simulink model "MOSSE_HDL_code_gen_final"  (Simulink 8.2)
settings: Solver=FixedStepDiscrete  SolverMode=SingleTasking  StartTime=0.0  StopTime=20*640*360  RelTol=1e-3
InitFcn:
  | %% DSPBuilder Start
  | alt_dspbuilder_update_model(bdroot)
  | %% DSPBuilder End
  | param
StopFcn:
  | % r = rcount.Data(:,:);
  | % w = wcount.Data(:,:);
  | % d = dout.Data(:,:);
  | % ir = read.Data(:,:);
  | % iw = write.Data(:,:);
  | % z = double([ir iw d r w]');
  | %logic_analyzer
values from neighbouring files (symbols this model uses):
  Gau = [4035 -3983 3832 -3589 3269 -2890 2472 -2039 1612 -1211 854 -553 ... (4096 elements, 1x4096)]    [Gauss_coeff.mat]    (also in param.m = reshape(conj(Gau'), 1, 4096))
undefined symbols (not defined in the file or in its folder): jet, psr, source_1, source_2, State_Machine, State_Transition_Table1, window_hann
libraries: allblocks_alteradspbuilder2 x182, hdldemolib x2, dspsigattribs x2, dspmtrx3 x2, visionsinks x1, visiontextngfix x1, dspvision x1
(part 1 of 3)
settings Model: FPTRunName=FPA_Reference  Creator=minimal  LastModifiedBy=Roma
settings DataIOCC: SignalLoggingSaveFormat=Dataset
settings OptimizationCC: ExpressionDepthLimit=128  OptimizeModelRefInitCode=on  LifeSpan=9
settings DebuggingCC: FcnCallInpInsideContextMsg=EnableAllAsError
settings HardwareCC: ProdHWDeviceType=ASIC/FPGA->ASIC/FPGA  TargetIntDivRoundTo=Zero  TargetEndianess=LittleEndian  TargetHWDeviceType=MATLAB Host  ProdEqTarget=off
settings RTWCC: SystemTargetFile=ert.tlc  TemplateMakefile=ert_default_tmf  Description=Embedded Coder  ProcessScript=ert_make_rtw_hook
settings CodeAppCC: IgnoreCustomStorageClasses=off
settings ERTTargetCC: CodeReplacementLibrary=ANSI_C  MultiwordLength=2048  GenerateSampleERTMain=on  ERTCustomFileTemplate=example_file_process.tlc  ConvertIfToSwitch=off  SuppressUnreachableDefaultCases=off

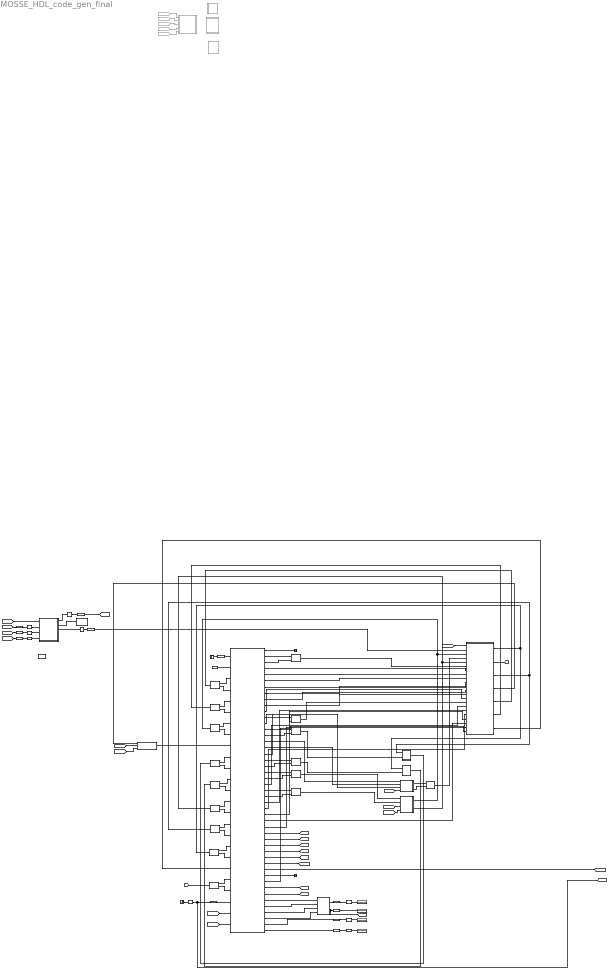
== system MOSSE_HDL_code_gen_final ==
  Complex to Real-Imag1 : allblocks_alteradspbuilder2/Complex to Real-Imag  BusType=Signed Integer  bwl=32  bwr=0  pipeline_display=0  allowFloatingPointOverride=on  logOutputs=off  logFile=E:\Project\AutoTracking\AutoTrack\Model\MOSSE_algorithm\MOSSE_simulink\tb_MOSSE_HDL_code_gen_final\MOSSE%5FHDL%5Fcode%5Fgen%5Ffinal_Complex+to+Real-Imag1%3A%3Aoutput%5Freal.fixedpointlog,E:\Project\AutoTracking\AutoTrack\Model\MOSSE_algorithm\MOSSE_simulink\tb_MOSSE_HDL_code_gen_final\MOSSE%5FHDL%5Fcode%5Fgen%5Ffinal_Complex+to+Real-Imag1%3A%3Aoutput%5Fimag.fixedpointlog,
  Complex to Real-Imag2 : allblocks_alteradspbuilder2/Complex to Real-Imag  BusType=Signed Integer  bwl=32  bwr=0  pipeline_display=0  allowFloatingPointOverride=on  logOutputs=off  logFile=E:\Project\AutoTracking\AutoTrack\Model\MOSSE_algorithm\MOSSE_simulink\tb_MOSSE_HDL_code_gen_final\MOSSE%5FHDL%5Fcode%5Fgen%5Ffinal_Complex+to+Real-Imag2%3A%3Aoutput%5Freal.fixedpointlog,E:\Project\AutoTracking\AutoTrack\Model\MOSSE_algorithm\MOSSE_simulink\tb_MOSSE_HDL_code_gen_final\MOSSE%5FHDL%5Fcode%5Fgen%5Ffinal_Complex+to+Real-Imag2%3A%3Aoutput%5Fimag.fixedpointlog,
  Complex to Real-Imag3 : allblocks_alteradspbuilder2/Complex to Real-Imag  BusType=Signed Integer  bwl=32  bwr=0  pipeline_display=0  allowFloatingPointOverride=on  logOutputs=off  logFile=E:\Project\AutoTracking\AutoTrack\Model\MOSSE_algorithm\MOSSE_simulink\tb_MOSSE_HDL_code_gen_final\MOSSE%5FHDL%5Fcode%5Fgen%5Ffinal_Complex+to+Real-Imag3%3A%3Aoutput%5Freal.fixedpointlog,E:\Project\AutoTracking\AutoTrack\Model\MOSSE_algorithm\MOSSE_simulink\tb_MOSSE_HDL_code_gen_final\MOSSE%5FHDL%5Fcode%5Fgen%5Ffinal_Complex+to+Real-Imag3%3A%3Aoutput%5Fimag.fixedpointlog,
  Complex to Real-Imag4 : allblocks_alteradspbuilder2/Complex to Real-Imag  BusType=Signed Integer  bwl=32  bwr=0  pipeline_display=0  allowFloatingPointOverride=on  logOutputs=off  logFile=E:\Project\AutoTracking\AutoTrack\Model\MOSSE_algorithm\MOSSE_simulink\tb_MOSSE_HDL_code_gen_final\MOSSE%5FHDL%5Fcode%5Fgen%5Ffinal_Complex+to+Real-Imag4%3A%3Aoutput%5Freal.fixedpointlog,E:\Project\AutoTracking\AutoTrack\Model\MOSSE_algorithm\MOSSE_simulink\tb_MOSSE_HDL_code_gen_final\MOSSE%5FHDL%5Fcode%5Fgen%5Ffinal_Complex+to+Real-Imag4%3A%3Aoutput%5Fimag.fixedpointlog,
  Complex to Real-Imag5 : allblocks_alteradspbuilder2/Complex to Real-Imag  BusType=Signed Integer  bwl=32  bwr=0  pipeline_display=0  allowFloatingPointOverride=on  logOutputs=off  logFile=E:\Project\AutoTracking\AutoTrack\Model\MOSSE_algorithm\MOSSE_simulink\tb_MOSSE_HDL_code_gen_final\MOSSE%5FHDL%5Fcode%5Fgen%5Ffinal_Complex+to+Real-Imag5%3A%3Aoutput%5Freal.fixedpointlog,E:\Project\AutoTracking\AutoTrack\Model\MOSSE_algorithm\MOSSE_simulink\tb_MOSSE_HDL_code_gen_final\MOSSE%5FHDL%5Fcode%5Fgen%5Ffinal_Complex+to+Real-Imag5%3A%3Aoutput%5Fimag.fixedpointlog,
  Complex to Real-Imag6 : allblocks_alteradspbuilder2/Complex to Real-Imag  BusType=Signed Integer  bwl=32  bwr=0  pipeline_display=0  allowFloatingPointOverride=on  logOutputs=off  logFile=E:\Project\AutoTracking\AutoTrack\Model\MOSSE_algorithm\MOSSE_simulink\tb_MOSSE_HDL_code_gen_final\MOSSE%5FHDL%5Fcode%5Fgen%5Ffinal_Complex+to+Real-Imag6%3A%3Aoutput%5Freal.fixedpointlog,E:\Project\AutoTracking\AutoTrack\Model\MOSSE_algorithm\MOSSE_simulink\tb_MOSSE_HDL_code_gen_final\MOSSE%5FHDL%5Fcode%5Fgen%5Ffinal_Complex+to+Real-Imag6%3A%3Aoutput%5Fimag.fixedpointlog,
  Complex to Real-Imag7 : allblocks_alteradspbuilder2/Complex to Real-Imag  BusType=Signed Integer  bwl=32  bwr=0  pipeline_display=0  allowFloatingPointOverride=on  logOutputs=off  logFile=E:\Project\AutoTracking\AutoTrack\Model\MOSSE_algorithm\MOSSE_simulink\tb_MOSSE_HDL_code_gen_final\MOSSE%5FHDL%5Fcode%5Fgen%5Ffinal_Complex+to+Real-Imag7%3A%3Aoutput%5Freal.fixedpointlog,E:\Project\AutoTracking\AutoTrack\Model\MOSSE_algorithm\MOSSE_simulink\tb_MOSSE_HDL_code_gen_final\MOSSE%5FHDL%5Fcode%5Fgen%5Ffinal_Complex+to+Real-Imag7%3A%3Aoutput%5Fimag.fixedpointlog,
  Complex to Real-Imag8 : allblocks_alteradspbuilder2/Complex to Real-Imag  BusType=Signed Integer  bwl=32  bwr=0  pipeline_display=0  allowFloatingPointOverride=on  logOutputs=off  logFile=E:\Project\AutoTracking\AutoTrack\Model\MOSSE_algorithm\MOSSE_simulink\tb_MOSSE_HDL_code_gen_final\MOSSE%5FHDL%5Fcode%5Fgen%5Ffinal_Complex+to+Real-Imag8%3A%3Aoutput%5Freal.fixedpointlog,E:\Project\AutoTracking\AutoTrack\Model\MOSSE_algorithm\MOSSE_simulink\tb_MOSSE_HDL_code_gen_final\MOSSE%5FHDL%5Fcode%5Fgen%5Ffinal_Complex+to+Real-Imag8%3A%3Aoutput%5Fimag.fixedpointlog,
  Complex to Real-Imag9 : allblocks_alteradspbuilder2/Complex to Real-Imag  BusType=Signed Integer  bwl=32  bwr=0  pipeline_display=0  allowFloatingPointOverride=on  logOutputs=off  logFile=E:\Project\AutoTracking\AutoTrack\Model\MOSSE_algorithm\MOSSE_simulink\tb_MOSSE_HDL_code_gen_final\MOSSE%5FHDL%5Fcode%5Fgen%5Ffinal_Complex+to+Real-Imag9%3A%3Aoutput%5Freal.fixedpointlog,E:\Project\AutoTracking\AutoTrack\Model\MOSSE_algorithm\MOSSE_simulink\tb_MOSSE_HDL_code_gen_final\MOSSE%5FHDL%5Fcode%5Fgen%5Ffinal_Complex+to+Real-Imag9%3A%3Aoutput%5Fimag.fixedpointlog,
  Constant : allblocks_alteradspbuilder2/Constant  mask_cst=1  BusType=Single Bit  bwl=8  bwr=0  roundMode=Truncate  satMode=Wrap  SpecifyClock=off  allowFloatingPointOverride=on  logOutputs=off  logFile=E:\Project\AutoTracking\AutoTrack\Model\MOSSE_algorithm\MOSSE_simulink\tb_MOSSE_HDL_code_gen_final\MOSSE%5FHDL%5Fcode%5Fgen%5Ffinal_Constant.fixedpointlog
  DSP_Buider_Alfa_blending_H1 : Subsystem
  DSP_Builder_Alfa_blending_H2 : Subsystem
  DSP_Builder_Compute_PSR : Subsystem  Commented=on
  DSP_Builder_Compute_Shift : Subsystem  Commented=on
  DSP_Builder_Divider Complex : Subsystem
  DSP_Builder_MEM_subsys : Subsystem
  DSP_Builder_Mult_complex : Subsystem
  DSP_Builder_PSR : Subsystem
  DSP_Builder_Smoothing_Window : Subsystem
  Data Type Conversion1 : DataTypeConversion  OutDataTypeStr=boolean
  Data Type Conversion19 : DataTypeConversion  OutDataTypeStr=int16
  Data Type Conversion2 : DataTypeConversion  OutDataTypeStr=int8
  Data Type Conversion3 : DataTypeConversion  OutDataTypeStr=int8
  Data Type Conversion5 : DataTypeConversion  OutDataTypeStr=boolean
  Data Type Conversion6 : DataTypeConversion  OutDataTypeStr=boolean
  Data Type Conversion7 : DataTypeConversion  OutDataTypeStr=uint16
  Delay2 : Delay  DelayLength=1  InitialCondition=0  SampleTime=1
  Delay3 : Delay  DelayLength=1  InitialCondition=0  SampleTime=1
  Display{1..4} (4 alike) : Display
  From38 : From  Commented=on  GotoTag=source_enb
  From39 : From  Commented=on  GotoTag=source1_enb
  From40 : From  Commented=on  GotoTag=source_control
  From41 : From  Commented=on  GotoTag=source_count_enb
  From42 : From  Commented=on  GotoTag=source_count_rst
  HDL Import : allblocks_alteradspbuilder2/HDLImport  entityName=HDL_CODER_Subsystem_import  inNames=reset clk_enable G_re G_im F_re F_im H2_re H2_im iPixel_image H1_alfa_re H1_alfa_im H2_alfa_re H2_alfa_im H1_re H1_im H1_p_re H1_p_im H2_p_re H2_p_im In12 iCorr_data_re iCorr_data_im enable_Tracking psr_check enable_write  inBwls=1 1 32 32 32 32 32 32 8 32 32 32 32 32 32 32 32 32 32 16 32 32 1 1 1  inBwrs="0  0  0  0  0  0  0  0  0  0  0  0  0  0  0  0  0  0  0  0  0  0  0  0  0"  inTypes=b b s s s s s s s s s s s s s s s s s s s s b b b  inDelayed="0  0  0  0  0  0  0  0  0  0  0  0  0  0  0  0  0  0  0  0  0  0  0  0  0"  outNames=ce_out oH2_re oH2_im wr_addr_H1_H2 we_H1_H2 wr_addr_G_F we_G_F addr_in_im rd_addr_H1_H2 rd_addr_G_F we_m oH1_re oH1_im oData1_re oData1_im Real_H1 Real_H2 Imag_H1 oData2_re oData2_im oF_re oF_im wr_addr_H oF_re_1 oF_im_1 we_H rd_addr_H RAM_data wr_addr_RAM_IFFT we_RAM_IFFT addr_memory_128x128 rst_win enb_win rst_gauss enb_gauss div_complex comp_shift_finish to_workspace_enb rd_addr_RAM_IFFT Dx Dy max_val mean_val tmp_val psr_reset psr_finish max_index  outBwls=1 32 32 12 1 12 1 14 12 12 1 32 32 32 32 32 32 32 32 32 32 32 12 32 32 1 12 16 12 1 14 1 1 1 1 1 1 1 12 8 8 16 16 44 1 1 13  outBwrs="0  0  0  0  0  0  0  0  0  0  0  0  0  0  0  0  0  0  0  0  0  0  0  0  0  0  0  0  0  0  0  0  0  0  0  0  0  0  0  0  0  0  0  0  0  0  0"  outTypes=b s s s b s b s s s b s s s s s s s s s s s s s s b s s s b s b b b b b b b s s s s s s b b s  xmlmapfile=C:\altera\13.0\quartus\dsp_builder\lib\SimgenCMap.xml  vofile=DSPBuilder_MOSSE_HDL_code_gen_final_import\HDL_CODER_Subsystem.vo  src_file=hdlsrc\HDL_CODER_subsys\MOSSE_HDL_final\Comp_Shift_code.v;hdlsrc\HDL_CODER_subsys\MOSSE_HDL_final\Comp_Shift_code_Subsys.v;hdlsrc\HDL_CODER_subsys\MOSSE_HDL_final\Complex_2_real_imag.v;hdlsrc\HDL_CODER_subsys\MOSSE_HDL_final\Compute_PSR_code.v;hdlsrc\HDL_CODER_subsys\MOSSE_HDL_final\FFT2D_System.v;hdlsrc\HDL_CODER_subsys\MOSSE_HDL_final\FFT2D_System_block.v;hdlsrc\HDL_CODER_subsys\MOSSE_HDL_final\HDL_CODER_Subsystem.v;hdlsrc\HDL_CODER_subsys\MOSSE_HDL_final\HDL_CODER_Subsystem_tc.v;hdlsrc\HDL_CODER_subsys\MOSSE_HDL_final\HDL_Streaming_FFT.v;hdlsrc\HDL_CODER_subsys\MOSSE_HDL_final\HDL_Streaming_FFT_Butterfly_DIF_Unit.v;hdlsrc\HDL_CODER_subsys\MOSSE_HDL_final\HDL_Streaming_FFT_Butterfly_DIF_Unit_Simple.v;hdlsrc\HDL_CODER_subsys\MOSSE_HDL_final\HDL_Streaming_FFT_stage_0.v;hdlsrc\HDL_CODER_subsys\MOSSE_HDL_final\HDL_Streaming_FFT_stage_1.v;hdlsrc\HDL_CODER_subsys\MOSSE_HDL_final\HDL_Streaming_FFT_stage_2.v;hdlsrc\HDL_CODER_subsys\MOSSE_HDL_final\HDL_Streaming_FFT_stage_3.v;hdlsrc\HDL_CODER_subsys\MOSSE_HDL_final\HDL_Streaming_FFT_stage_4.v;hdlsrc\HDL_CODER_subsys\MOSSE_HDL_final\HDL_Streaming_FFT_stage_5.v;hdlsrc\HDL_CODER_subsys\MOSSE_HDL_final\HDL_Streaming_FFT_stage_end.v;hdlsrc\HDL_CODER_subsys\MOSSE_HDL_final\HDL_Streaming_FFT_stage_init.v;hdlsrc\HDL_CODER_subsys\MOSSE_HDL_final\HDL_Streaming_FFT_stage_init_RAM.v;hdlsrc\HDL_CODER_subsys\MOSSE_HDL_final\IFFT_MUX.v;hdlsrc\HDL_CODER_subsys\MOSSE_HDL_final\IFFT2D.v;hdlsrc\HDL_CODER_subsys\MOSSE_HDL_final\im_RAM_STM.v;hdlsrc\HDL_CODER_subsys\MOSSE_HDL_final\Main_State_Machine.v;hdlsrc\HDL_CODER_subsys\MOSSE_HDL_final\Memory_Counter.v;hdlsrc\HDL_CODER_subsys\MOSSE_HDL_final\Memory_Counter_Subsys.v;hdlsrc\HDL_CODER_subsys\MOSSE_HDL_final\MOSSE_SM.v;hdlsrc\HDL_CODER_subsys\MOSSE_HDL_final\Mux_Mult.v;hdlsrc\HDL_CODER_subsys\MOSSE_HDL_final\Mux_system.v;hdlsrc\HDL_CODER_subsys\MOSSE_HDL_final\psr_code_subsys.v;hdlsrc\HDL_CODER_subsys\MOSSE_HDL_final\R_RAM.v;hdlsrc\HDL_CODER_subsys\MOSSE_HDL_final\Read_Write_patched_2.v;hdlsrc\HDL_CODER_subsys\MOSSE_HDL_final\Read_Write_SM1_patched_1.v;hdlsrc\HDL_CODER_subsys\MOSSE_HDL_final\Read_Write_SM1_patched_2.v;hdlsrc\HDL_CODER_subsys\MOSSE_HDL_final\Read_Write_SM1_patched_2_block.v;hdlsrc\HDL_CODER_subsys\MOSSE_HDL_final\Read_Write_SM1_patched_2_block1.v;hdlsrc\HDL_CODER_subsys\MOSSE_HDL_final\Read_Write_SM6.v;hdlsrc\HDL_CODER_subsys\MOSSE_HDL_final\SimpDualPortRAM_Inst0.v;hdlsrc\HDL_CODER_subsys\MOSSE_HDL_final\SimpDualPortRAM_Inst1.v;hdlsrc\HDL_CODER_subsys\MOSSE_HDL_final\SimpleDualPortRAM_64x48b.v;hdlsrc\HDL_CODER_subsys\MOSSE_HDL_final\SimpleDualPortRAM_4096x48b.v;hdlsrc\HDL_CODER_subsys\MOSSE_HDL_final\SimpleDualPortRAM_4096x48b_block.v;hdlsrc\HDL_CODER_subsys\MOSSE_HDL_final\SM_H_RAM.v;hdlsrc\HDL_CODER_subsys\MOSSE_HDL_final\SM_memory.v;hdlsrc\HDL_CODER_subsys\MOSSE_HDL_final\SM_memory_H1_H2.v;hdlsrc\HDL_CODER_subsys\MOSSE_HDL_final\SM_RAM_IFFT_res.v;hdlsrc\HDL_CODER_subsys\MOSSE_HDL_final\SM_temp_G_F.v;hdlsrc\HDL_CODER_subsys\MOSSE_HDL_final\State_Machine_FFT2.v;hdlsrc\HDL_CODER_subsys\MOSSE_HDL_final\Transpone_Counter.v;  TopLevelName=HDL_CODER_Subsystem  UseQPF=0  n_input_port=25  n_output_port=47  array_clocks=clk  use_systemC_model=off  is_megacore=off  use_dynamic_feedthrough_data=off  use_alphabetical_port_ordering=off  allowFloatingPointOverride=off
  IFFT_res : hdldemolib/Single Port RAM  Commented=on  ram_size=12  dout_type=New data
  Input_image : allblocks_alteradspbuilder2/Input  iofile=E:\Project\AutoTracking\AutoTrack\Model\MOSSE_algorithm\MOSSE_simulink\tb_MOSSE_HDL_code_gen_final\MOSSE%5FHDL%5Fcode%5Fgen%5Ffinal_Input%5Fimage.salt  BusType=Unsigned Integer  bwl=8  bwr=0  SpecifyClock=off  PORTTYPE=Input  externalType=Inferred  allowFloatingPointOverride=on  logOutputs=off
  Real-Imag to Complex2 : allblocks_alteradspbuilder2/Real-Imag to Complex  BusType=Signed Integer  bwl=32  bwr=0  pipeline_display=0  allowFloatingPointOverride=on  logOutputs=off  logFile=E:\Project\AutoTracking\AutoTrack\Model\MOSSE_algorithm\MOSSE_simulink\tb_MOSSE_HDL_code_gen_final\MOSSE%5FHDL%5Fcode%5Fgen%5Ffinal_Real-Imag+to+Complex2.fixedpointlog
  Real-Imag to Complex3 : allblocks_alteradspbuilder2/Real-Imag to Complex  BusType=Signed Integer  bwl=32  bwr=0  pipeline_display=0  allowFloatingPointOverride=on  logOutputs=off  logFile=E:\Project\AutoTracking\AutoTrack\Model\MOSSE_algorithm\MOSSE_simulink\tb_MOSSE_HDL_code_gen_final\MOSSE%5FHDL%5Fcode%5Fgen%5Ffinal_Real-Imag+to+Complex3.fixedpointlog
  Real-Imag to Complex4 : allblocks_alteradspbuilder2/Real-Imag to Complex  BusType=Signed Integer  bwl=32  bwr=0  pipeline_display=0  allowFloatingPointOverride=on  logOutputs=off  logFile=E:\Project\AutoTracking\AutoTrack\Model\MOSSE_algorithm\MOSSE_simulink\tb_MOSSE_HDL_code_gen_final\MOSSE%5FHDL%5Fcode%5Fgen%5Ffinal_Real-Imag+to+Complex4.fixedpointlog
  Real-Imag to Complex5 : allblocks_alteradspbuilder2/Real-Imag to Complex  BusType=Signed Integer  bwl=32  bwr=0  pipeline_display=0  allowFloatingPointOverride=on  logOutputs=off  logFile=E:\Project\AutoTracking\AutoTrack\Model\MOSSE_algorithm\MOSSE_simulink\tb_MOSSE_HDL_code_gen_final\MOSSE%5FHDL%5Fcode%5Fgen%5Ffinal_Real-Imag+to+Complex5.fixedpointlog
  Real-Imag to Complex6 : allblocks_alteradspbuilder2/Real-Imag to Complex  BusType=Signed Integer  bwl=32  bwr=0  pipeline_display=0  allowFloatingPointOverride=on  logOutputs=off  logFile=E:\Project\AutoTracking\AutoTrack\Model\MOSSE_algorithm\MOSSE_simulink\tb_MOSSE_HDL_code_gen_final\MOSSE%5FHDL%5Fcode%5Fgen%5Ffinal_Real-Imag+to+Complex6.fixedpointlog
  Real-Imag to Complex7 : allblocks_alteradspbuilder2/Real-Imag to Complex  BusType=Signed Integer  bwl=32  bwr=0  pipeline_display=0  allowFloatingPointOverride=on  logOutputs=off  logFile=E:\Project\AutoTracking\AutoTrack\Model\MOSSE_algorithm\MOSSE_simulink\tb_MOSSE_HDL_code_gen_final\MOSSE%5FHDL%5Fcode%5Fgen%5Ffinal_Real-Imag+to+Complex7.fixedpointlog
  Real-Imag to Complex8 : allblocks_alteradspbuilder2/Real-Imag to Complex  BusType=Signed Integer  bwl=32  bwr=0  pipeline_display=0  allowFloatingPointOverride=on  logOutputs=off  logFile=E:\Project\AutoTracking\AutoTrack\Model\MOSSE_algorithm\MOSSE_simulink\tb_MOSSE_HDL_code_gen_final\MOSSE%5FHDL%5Fcode%5Fgen%5Ffinal_Real-Imag+to+Complex8.fixedpointlog
  Signal Compiler : allblocks_alteradspbuilder2/Signal Compiler  DeviceFamily=Cyclone IV E  DeviceName=AUTO  EnableSignalTap=off  SignalTapDepth=128  UseBoardBlock=off  StpUseDefaultClock=on  StpClock=Clock  ExportDir=C:\Users\Roma\Documents
  Source : Subsystem  Commented=on
  Step : Step  Before=1  After=0  SampleTime=0
  Step1 : Step  SampleTime=0
  Terminator1 : Terminator
  Terminator2 : Terminator
  Video Viewer2 : visionsinks/Video Viewer  inputType=Obsolete7b  imagePorts=One multidimensional signal  useColorMap=off  colormapValue=jet(256)  specRange=off  minInputVal=0  maxInputVal=255  FigPos=[713 697 410 300]  AxisZoom=on  trueSizedOnce=off  OpenAtMdlStart=on  DefaultConfigurationName=vipscopes.VideoViewerScopeCfg
  Video_TestBench1 : Subsystem
  comp_shift_finish : allblocks_alteradspbuilder2/Output  iofile=E:\Project\AutoTracking\AutoTrack\Model\MOSSE_algorithm\MOSSE_simulink\tb_MOSSE_HDL_code_gen_final\MOSSE%5FHDL%5Fcode%5Fgen%5Ffinal_comp%5Fshift%5Ffinish.capture  BusType=Single Bit  bwl=8  bwr=0  externalType=Simulink Fixed Point Type  PORTTYPE=Output  allowFloatingPointOverride=on  logOutputs=off
  dx : allblocks_alteradspbuilder2/Output  iofile=E:\Project\AutoTracking\AutoTrack\Model\MOSSE_algorithm\MOSSE_simulink\tb_MOSSE_HDL_code_gen_final\MOSSE%5FHDL%5Fcode%5Fgen%5Ffinal_dx.capture  BusType=Signed Integer  bwl=8  bwr=0  externalType=Simulink Fixed Point Type  PORTTYPE=Output  allowFloatingPointOverride=on  logOutputs=off
  dy : allblocks_alteradspbuilder2/Output  iofile=E:\Project\AutoTracking\AutoTrack\Model\MOSSE_algorithm\MOSSE_simulink\tb_MOSSE_HDL_code_gen_final\MOSSE%5FHDL%5Fcode%5Fgen%5Ffinal_dy.capture  BusType=Signed Integer  bwl=8  bwr=0  externalType=Simulink Fixed Point Type  PORTTYPE=Output  allowFloatingPointOverride=on  logOutputs=off
  enable_tracking : allblocks_alteradspbuilder2/Input  iofile=E:\Project\AutoTracking\AutoTrack\Model\MOSSE_algorithm\MOSSE_simulink\tb_MOSSE_HDL_code_gen_final\MOSSE%5FHDL%5Fcode%5Fgen%5Ffinal_enable%5Ftracking.salt  BusType=Single Bit  bwl=8  bwr=0  SpecifyClock=off  PORTTYPE=Input  externalType=Inferred  allowFloatingPointOverride=on  logOutputs=off
  enable_write : allblocks_alteradspbuilder2/Input  iofile=E:\Project\AutoTracking\AutoTrack\Model\MOSSE_algorithm\MOSSE_simulink\tb_MOSSE_HDL_code_gen_final\MOSSE%5FHDL%5Fcode%5Fgen%5Ffinal_enable%5Fwrite.salt  BusType=Single Bit  bwl=8  bwr=0  SpecifyClock=off  PORTTYPE=Input  externalType=Inferred  allowFloatingPointOverride=on  logOutputs=off
  max_index : allblocks_alteradspbuilder2/Output  iofile=E:\Project\AutoTracking\AutoTrack\Model\MOSSE_algorithm\MOSSE_simulink\tb_MOSSE_HDL_code_gen_final\MOSSE%5FHDL%5Fcode%5Fgen%5Ffinal_max%5Findex.capture  BusType=Unsigned Integer  bwl=13  bwr=0  externalType=Simulink Fixed Point Type  PORTTYPE=Output  allowFloatingPointOverride=on  logOutputs=off
  psr : allblocks_alteradspbuilder2/Output  iofile=E:\Project\AutoTracking\AutoTrack\Model\MOSSE_algorithm\MOSSE_simulink\tb_MOSSE_HDL_code_gen_final\MOSSE%5FHDL%5Fcode%5Fgen%5Ffinal_psr.capture  BusType=Signed Integer  bwl=16  bwr=0  externalType=Simulink Fixed Point Type  PORTTYPE=Output  allowFloatingPointOverride=on  logOutputs=off
  psr_check : allblocks_alteradspbuilder2/Output  iofile=E:\Project\AutoTracking\AutoTrack\Model\MOSSE_algorithm\MOSSE_simulink\tb_MOSSE_HDL_code_gen_final\MOSSE%5FHDL%5Fcode%5Fgen%5Ffinal_psr%5Fcheck.capture  BusType=Single Bit  bwl=16  bwr=0  externalType=Simulink Fixed Point Type  PORTTYPE=Output  allowFloatingPointOverride=on  logOutputs=off
  psr_finish : allblocks_alteradspbuilder2/Output  iofile=E:\Project\AutoTracking\AutoTrack\Model\MOSSE_algorithm\MOSSE_simulink\tb_MOSSE_HDL_code_gen_final\MOSSE%5FHDL%5Fcode%5Fgen%5Ffinal_psr%5Ffinish.capture  BusType=Single Bit  bwl=16  bwr=0  externalType=Simulink Fixed Point Type  PORTTYPE=Output  allowFloatingPointOverride=on  logOutputs=off
  reset : allblocks_alteradspbuilder2/Input  iofile=E:\Project\AutoTracking\AutoTrack\Model\MOSSE_algorithm\MOSSE_simulink\tb_MOSSE_HDL_code_gen_final\MOSSE%5FHDL%5Fcode%5Fgen%5Ffinal_reset.salt  BusType=Single Bit  bwl=8  bwr=0  SpecifyClock=off  PORTTYPE=Input  externalType=Inferred  allowFloatingPointOverride=on  logOutputs=off
  wires:
  From40/1 -> Source/1(source_control)
  From38/1 -> Source/2(source_enb)
  From42/1 -> Source/3(source_count_rst)
  From41/1 -> Source/4(source_count_enb)
  From39/1 -> Source/5(source1_enb)
  DSP_Builder_Divider Complex/2(Im_r) -> Real-Imag to Complex5/2
  DSP_Builder_Divider Complex/1(Re_r) -> Real-Imag to Complex5/1
  [rst_win] -> DSP_Builder_Smoothing_Window/2(rst)
  [enb_win] -> DSP_Builder_Smoothing_Window/3(enb)
  [div_complex_aclr] -> DSP_Builder_Divider Complex/4(aclr_i)
  [rst_gauss] -> DSP_Builder_Mult_complex/3(rst)
  [enb_gauss] -> DSP_Builder_Mult_complex/4(enb)
  DSP_Builder_Mult_complex/1(H2) -> DSP_Builder_MEM_subsys/3(wr_din_F_RAM), Complex to Real-Imag3/1
  DSP_Builder_Mult_complex/2(H1) -> DSP_Builder_MEM_subsys/5(wr_din_G_RAM), Complex to Real-Imag1/1
  DSP_Builder_Smoothing_Window/1(opixel) -> HDL Import/9
  DSP_Buider_Alfa_blending_H1/1(H) -> Complex to Real-Imag8/1
  DSP_Builder_Alfa_blending_H2/1(H) -> Complex to Real-Imag9/1
  [Corr] -> Complex to Real-Imag7/1
  Data Type Conversion5/1 -> [enable_tracking], enable_tracking/1
  [psr_check] -> HDL Import/24
  Real-Imag to Complex6/1 -> DSP_Buider_Alfa_blending_H1/2(H_n)
  HDL Import/16 -> DSP_Builder_Divider Complex/1(Re_a)
  HDL Import/17 -> DSP_Builder_Divider Complex/2(Re_b)
  HDL Import/18 -> DSP_Builder_Divider Complex/3(Im_a)
  Real-Imag to Complex2/1 -> DSP_Builder_Alfa_blending_H2/2(H_n)
  HDL Import/37 -> [comp_shift_finish]
  [comp_shift_finish] -> comp_shift_finish/1
  Video_TestBench1/2(video_viewer) -> Video Viewer2/1
  [enable_write] -> HDL Import/25
  Video_TestBench1/1(enable_write) -> Delay2/1
  Delay2/1 -> enable_write/1
  Video_TestBench1/3(serialized_data) -> Delay3/1
  DSP_Builder_MEM_subsys/3(rd_dout_H1_RAM) -> DSP_Buider_Alfa_blending_H1/1(H_p), Complex to Real-Imag4/1
  DSP_Builder_MEM_subsys/1(rd_dout_H2_RAM) -> DSP_Builder_Alfa_blending_H2/1(H_p), Complex to Real-Imag2/1
  [mem_addr] -> DSP_Builder_MEM_subsys/1(rd_addr_Ext_im_RAM)
  Input_image/1 -> DSP_Builder_MEM_subsys/2(wr_din_Ext_im_RAM)
  Real-Imag to Complex5/1 -> DSP_Builder_MEM_subsys/4(wr_din_H_RAM)
  Real-Imag to Complex8/1 -> DSP_Builder_MEM_subsys/6(wr_din_H2_RAM)
  HDL Import/4 -> DSP_Builder_MEM_subsys/7(wr_addr_H1_H2_RAM)
  HDL Import/5 -> DSP_Builder_MEM_subsys/8(wr_en_H1_H2_RAM)
  HDL Import/6 -> DSP_Builder_MEM_subsys/9(wr_addr_G_F_RAM)
  HDL Import/7 -> DSP_Builder_MEM_subsys/10(wr_en_G_F_RAM)
  HDL Import/8 -> DSP_Builder_MEM_subsys/11(wr_addr_Ext_im_RAM)
  HDL Import/9 -> DSP_Builder_MEM_subsys/12(rd_addr_H1_H2_RAM)
  HDL Import/10 -> DSP_Builder_MEM_subsys/13(rd_addr_G_F_RAM)
  HDL Import/11 -> DSP_Builder_MEM_subsys/14(wr_en_Ext_im_RAM)
  Real-Imag to Complex7/1 -> DSP_Builder_MEM_subsys/15(wr_din_H1_RAM)
  HDL Import/23 -> DSP_Builder_MEM_subsys/16(wr_addr_H_RAM)
  HDL Import/26 -> DSP_Builder_MEM_subsys/17(wr_en_H_RAM)
  HDL Import/27 -> DSP_Builder_MEM_subsys/18(rd_addr_H_RAM)
  HDL Import/28 -> DSP_Builder_MEM_subsys/19(wr_din_IFFT_res_RAM)
  HDL Import/29 -> DSP_Builder_MEM_subsys/20(wr_addr_IFFT_res_RAM)
  HDL Import/30 -> DSP_Builder_MEM_subsys/21(wr_en_IFFT_res_RAM)
  HDL Import/39 -> DSP_Builder_MEM_subsys/22(rd_addr_IFFT_res_RAM)
  DSP_Builder_MEM_subsys/2(rd_dout_H_RAM) -> [Corr]
  DSP_Builder_MEM_subsys/4(rd_dout_Ext_im_RAM) -> DSP_Builder_Smoothing_Window/1(ipixel)
  DSP_Builder_MEM_subsys/5(rd_dout_G_RAM) -> Complex to Real-Imag5/1
  DSP_Builder_MEM_subsys/6(rd_dout_F_RAM) -> Complex to Real-Imag6/1
  DSP_Builder_MEM_subsys/7(rd_dout_IFFT_res_RAM) -> HDL Import/20
  HDL Import/42 -> DSP_Builder_PSR/1(max)
  HDL Import/43 -> DSP_Builder_PSR/2(mean)
  HDL Import/44 -> DSP_Builder_PSR/3(tmp)
  HDL Import/40 -> [dx]
  HDL Import/41 -> [dy]
  HDL Import/31 -> [mem_addr]
  HDL Import/32 -> [rst_win]
  HDL Import/33 -> [enb_win]
  HDL Import/34 -> [rst_gauss]
  HDL Import/35 -> [enb_gauss]
  HDL Import/36 -> [div_complex_aclr]
  HDL Import/19 -> Real-Imag to Complex2/1
  HDL Import/20 -> Real-Imag to Complex2/2
  HDL Import/21 -> Real-Imag to Complex3/1
  HDL Import/22 -> Real-Imag to Complex3/2
  HDL Import/24 -> Real-Imag to Complex4/1
  HDL Import/25 -> Real-Imag to Complex4/2
  HDL Import/14 -> Real-Imag to Complex6/1
  HDL Import/15 -> Real-Imag to Complex6/2
  HDL Import/12 -> Real-Imag to Complex7/1
  HDL Import/13 -> Real-Imag to Complex7/2
  HDL Import/2 -> Real-Imag to Complex8/1
  HDL Import/3 -> Real-Imag to Complex8/2
  Complex to Real-Imag3/1 -> HDL Import/7
  Complex to Real-Imag3/2 -> HDL Import/8
  Complex to Real-Imag1/1 -> HDL Import/14
  Complex to Real-Imag1/2 -> HDL Import/15
  Complex to Real-Imag2/1 -> HDL Import/18
  Complex to Real-Imag2/2 -> HDL Import/19
  Complex to Real-Imag4/1 -> HDL Import/16
  Complex to Real-Imag4/2 -> HDL Import/17
  Complex to Real-Imag5/1 -> HDL Import/3
  Complex to Real-Imag5/2 -> HDL Import/4
  Complex to Real-Imag6/2 -> HDL Import/6
  Complex to Real-Imag6/1 -> HDL Import/5
  Complex to Real-Imag7/1 -> HDL Import/21
  Complex to Real-Imag7/2 -> HDL Import/22
  Complex to Real-Imag8/1 -> HDL Import/10
  Complex to Real-Imag8/2 -> HDL Import/11
  Complex to Real-Imag9/1 -> HDL Import/12
  Complex to Real-Imag9/2 -> HDL Import/13
  reset/1 -> HDL Import/1
  Constant/1 -> HDL Import/2
  HDL Import/1 -> Terminator1/1
  [dx] -> dx/1
  [dy] -> dy/1
  Delay3/1 -> Input_image/1
  enable_write/1 -> [enable_write]
  HDL Import/38 -> Terminator2/1
  [enable_tracking] -> Video_TestBench1/1(en)
  comp_shift_finish/1 -> Data Type Conversion1/1
  Data Type Conversion1/1 -> Video_TestBench1/4(comp_shift_finish)
  dx/1 -> Data Type Conversion2/1
  dy/1 -> Data Type Conversion3/1
  Data Type Conversion2/1 -> Video_TestBench1/2(dx)
  Data Type Conversion3/1 -> Video_TestBench1/3(dy)
  Real-Imag to Complex3/1 -> DSP_Builder_Mult_complex/1(F*)
  Real-Imag to Complex4/1 -> DSP_Builder_Mult_complex/2(F)
  Data Type Conversion19/1 -> Display1/1
  DSP_Builder_PSR/1(psr) -> psr/1
  DSP_Builder_PSR/2(psr_check) -> [psr_check], psr_check/1
  HDL Import/45 -> DSP_Builder_PSR/4(psr_reset)
  Step/1 -> reset/1
  enable_tracking/1 -> HDL Import/23
  Step1/1 -> Data Type Conversion5/1
  psr/1 -> Data Type Conversion19/1
  HDL Import/46 -> psr_finish/1
  psr_finish/1 -> Data Type Conversion6/1
  Data Type Conversion6/1 -> Display2/1
  HDL Import/47 -> max_index/1
  max_index/1 -> Data Type Conversion7/1
  Data Type Conversion7/1 -> Display3/1
  psr_check/1 -> Display4/1

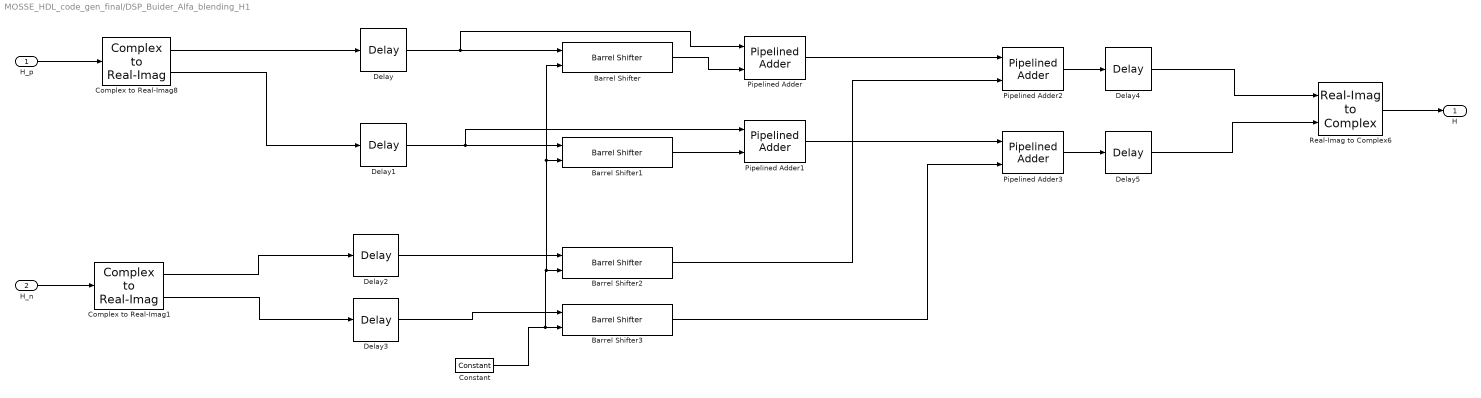
== system MOSSE_HDL_code_gen_final/DSP_Buider_Alfa_blending_H1 ==
  H_p : Inport
  H_n : Inport  Port=2
  Barrel Shifter : allblocks_alteradspbuilder2/Barrel Shifter  BusType=Signed Integer  bwl=32  bwr=8  pipeline=off  infer_distance=off  distance_length=3  ShiftDirection=Shift right  use_ena=off  use_aclr=off  UseDedicatedCircuitry=off  pipeline_display=0  allowFloatingPointOverride=on  logOutputs=off  logFile=E:\Project\AutoTracking\model\MOSSE_work\MOSSE_model\test\tb_MOSSE_HDL_code_gen_final\MOSSE%5FHDL%5Fcode%5Fgen%5Ffinal_DSP%5FBuider%5FAlfa%5Fblending%5FH1_Barrel+Shifter.fixedpointlog
  Barrel Shifter1 : allblocks_alteradspbuilder2/Barrel Shifter  BusType=Signed Integer  bwl=32  bwr=8  pipeline=off  infer_distance=off  distance_length=3  ShiftDirection=Shift right  use_ena=off  use_aclr=off  UseDedicatedCircuitry=off  pipeline_display=0  allowFloatingPointOverride=on  logOutputs=off  logFile=E:\Project\AutoTracking\model\MOSSE_work\MOSSE_model\test\tb_MOSSE_HDL_code_gen_final\MOSSE%5FHDL%5Fcode%5Fgen%5Ffinal_DSP%5FBuider%5FAlfa%5Fblending%5FH1_Barrel+Shifter1.fixedpointlog
  Barrel Shifter2 : allblocks_alteradspbuilder2/Barrel Shifter  BusType=Signed Integer  bwl=32  bwr=8  pipeline=off  infer_distance=off  distance_length=3  ShiftDirection=Shift right  use_ena=off  use_aclr=off  UseDedicatedCircuitry=off  pipeline_display=0  allowFloatingPointOverride=on  logOutputs=off  logFile=E:\Project\AutoTracking\model\MOSSE_work\MOSSE_model\test\tb_MOSSE_HDL_code_gen_final\MOSSE%5FHDL%5Fcode%5Fgen%5Ffinal_DSP%5FBuider%5FAlfa%5Fblending%5FH1_Barrel+Shifter2.fixedpointlog
  Barrel Shifter3 : allblocks_alteradspbuilder2/Barrel Shifter  BusType=Signed Integer  bwl=32  bwr=8  pipeline=off  infer_distance=off  distance_length=3  ShiftDirection=Shift right  use_ena=off  use_aclr=off  UseDedicatedCircuitry=off  pipeline_display=0  allowFloatingPointOverride=on  logOutputs=off  logFile=E:\Project\AutoTracking\model\MOSSE_work\MOSSE_model\test\tb_MOSSE_HDL_code_gen_final\MOSSE%5FHDL%5Fcode%5Fgen%5Ffinal_DSP%5FBuider%5FAlfa%5Fblending%5FH1_Barrel+Shifter3.fixedpointlog
  Complex to Real-Imag1 : allblocks_alteradspbuilder2/Complex to Real-Imag  BusType=Signed Integer  bwl=32  bwr=0  pipeline_display=0  allowFloatingPointOverride=on  logOutputs=off  logFile=E:\Project\AutoTracking\model\MOSSE_work\MOSSE_model\test\tb_MOSSE_HDL_code_gen_final\MOSSE%5FHDL%5Fcode%5Fgen%5Ffinal_DSP%5FBuider%5FAlfa%5Fblending%5FH1_Complex+to+Real-Imag1%3A%3Aoutput%5Freal.fixedpointlog,E:\Project\AutoTracking\model\MOSSE_work\MOSSE_model\test\tb_MOSSE_HDL_code_gen_final\MOSSE%5FHDL%5Fcode%5Fgen%5Ffinal_DSP%5FBuider%5FAlfa%5Fblending%5FH1_Complex+to+Real-Imag1%3A%3Aoutput%5Fimag.fixedpointlog,
  Complex to Real-Imag8 : allblocks_alteradspbuilder2/Complex to Real-Imag  BusType=Signed Integer  bwl=32  bwr=0  pipeline_display=0  allowFloatingPointOverride=on  logOutputs=off  logFile=E:\Project\AutoTracking\model\MOSSE_work\MOSSE_model\test\tb_MOSSE_HDL_code_gen_final\MOSSE%5FHDL%5Fcode%5Fgen%5Ffinal_DSP%5FBuider%5FAlfa%5Fblending%5FH1_Complex+to+Real-Imag8%3A%3Aoutput%5Freal.fixedpointlog,E:\Project\AutoTracking\model\MOSSE_work\MOSSE_model\test\tb_MOSSE_HDL_code_gen_final\MOSSE%5FHDL%5Fcode%5Fgen%5Ffinal_DSP%5FBuider%5FAlfa%5Fblending%5FH1_Complex+to+Real-Imag8%3A%3Aoutput%5Fimag.fixedpointlog,
  Constant : allblocks_alteradspbuilder2/Constant  mask_cst=K_shift  BusType=Unsigned Integer  bwl=3  bwr=0  roundMode=Truncate  satMode=Wrap  SpecifyClock=off  allowFloatingPointOverride=on  logOutputs=off  logFile=E:\Project\AutoTracking\model\MOSSE_work\MOSSE_model\test\tb_MOSSE_HDL_code_gen_final\MOSSE%5FHDL%5Fcode%5Fgen%5Ffinal_DSP%5FBuider%5FAlfa%5Fblending%5FH1_Constant.fixedpointlog
  Delay : allblocks_alteradspbuilder2/Delay  pipeline=1  pipeline_display=1  ClockPhase=1  use_ena=off  use_sclr=off  allowFloatingPointOverride=on  logOutputs=off  logFile=E:\Project\AutoTracking\model\MOSSE_work\MOSSE_model\test\tb_MOSSE_HDL_code_gen_final\MOSSE%5FHDL%5Fcode%5Fgen%5Ffinal_DSP%5FBuider%5FAlfa%5Fblending%5FH1_Delay.fixedpointlog  use_init=off  reset_value=1
  Delay1 : allblocks_alteradspbuilder2/Delay  pipeline=1  pipeline_display=1  ClockPhase=1  use_ena=off  use_sclr=off  allowFloatingPointOverride=on  logOutputs=off  logFile=E:\Project\AutoTracking\model\MOSSE_work\MOSSE_model\test\tb_MOSSE_HDL_code_gen_final\MOSSE%5FHDL%5Fcode%5Fgen%5Ffinal_DSP%5FBuider%5FAlfa%5Fblending%5FH1_Delay1.fixedpointlog  use_init=off  reset_value=1
  Delay2 : allblocks_alteradspbuilder2/Delay  pipeline=1  pipeline_display=1  ClockPhase=1  use_ena=off  use_sclr=off  allowFloatingPointOverride=on  logOutputs=off  logFile=E:\Project\AutoTracking\model\MOSSE_work\MOSSE_model\test\tb_MOSSE_HDL_code_gen_final\MOSSE%5FHDL%5Fcode%5Fgen%5Ffinal_DSP%5FBuider%5FAlfa%5Fblending%5FH1_Delay2.fixedpointlog  use_init=off  reset_value=1
  Delay3 : allblocks_alteradspbuilder2/Delay  pipeline=1  pipeline_display=1  ClockPhase=1  use_ena=off  use_sclr=off  allowFloatingPointOverride=on  logOutputs=off  logFile=E:\Project\AutoTracking\model\MOSSE_work\MOSSE_model\test\tb_MOSSE_HDL_code_gen_final\MOSSE%5FHDL%5Fcode%5Fgen%5Ffinal_DSP%5FBuider%5FAlfa%5Fblending%5FH1_Delay3.fixedpointlog  use_init=off  reset_value=1
  Delay4 : allblocks_alteradspbuilder2/Delay  pipeline=1  pipeline_display=1  ClockPhase=1  use_ena=off  use_sclr=off  allowFloatingPointOverride=on  logOutputs=off  logFile=E:\Project\AutoTracking\model\MOSSE_work\MOSSE_model\test\tb_MOSSE_HDL_code_gen_final\MOSSE%5FHDL%5Fcode%5Fgen%5Ffinal_DSP%5FBuider%5FAlfa%5Fblending%5FH1_Delay4.fixedpointlog  use_init=off  reset_value=1
  Delay5 : allblocks_alteradspbuilder2/Delay  pipeline=1  pipeline_display=1  ClockPhase=1  use_ena=off  use_sclr=off  allowFloatingPointOverride=on  logOutputs=off  logFile=E:\Project\AutoTracking\model\MOSSE_work\MOSSE_model\test\tb_MOSSE_HDL_code_gen_final\MOSSE%5FHDL%5Fcode%5Fgen%5Ffinal_DSP%5FBuider%5FAlfa%5Fblending%5FH1_Delay5.fixedpointlog  use_init=off  reset_value=1
  Pipelined Adder : allblocks_alteradspbuilder2/Pipelined Adder  BusType=Signed Integer  bwl=32  bwr=0  pipeline=0  pipeline_display=0  AddSubDirection=SUB  use_cin=off  use_ovl=off  use_addsub=off  use_ena=off  use_aclr=off  or_aclr_inputs=on
  Pipelined Adder1 : allblocks_alteradspbuilder2/Pipelined Adder  BusType=Signed Integer  bwl=32  bwr=0  pipeline=0  pipeline_display=0  AddSubDirection=SUB  use_cin=off  use_ovl=off  use_addsub=off  use_ena=off  use_aclr=off  or_aclr_inputs=on
  Pipelined Adder2 : allblocks_alteradspbuilder2/Pipelined Adder  BusType=Signed Integer  bwl=32  bwr=0  pipeline=0  pipeline_display=0  AddSubDirection=ADD  use_cin=off  use_ovl=off  use_addsub=off  use_ena=off  use_aclr=off  or_aclr_inputs=on
  Pipelined Adder3 : allblocks_alteradspbuilder2/Pipelined Adder  BusType=Signed Integer  bwl=32  bwr=0  pipeline=0  pipeline_display=0  AddSubDirection=ADD  use_cin=off  use_ovl=off  use_addsub=off  use_ena=off  use_aclr=off  or_aclr_inputs=on
  Real-Imag to Complex6 : allblocks_alteradspbuilder2/Real-Imag to Complex  BusType=Signed Integer  bwl=32  bwr=0  pipeline_display=0  allowFloatingPointOverride=on  logOutputs=off  logFile=E:\Project\AutoTracking\model\MOSSE_work\MOSSE_model\test\tb_MOSSE_HDL_code_gen_final\MOSSE%5FHDL%5Fcode%5Fgen%5Ffinal_DSP%5FBuider%5FAlfa%5Fblending%5FH1_Real-Imag+to+Complex6.fixedpointlog
  H : Outport
  wires:
  Pipelined Adder/1 -> Pipelined Adder2/1
  Barrel Shifter/1 -> Pipelined Adder/2
  Barrel Shifter2/1 -> Pipelined Adder2/2
  Barrel Shifter3/1 -> Pipelined Adder3/2
  Pipelined Adder1/1 -> Pipelined Adder3/1
  Barrel Shifter1/1 -> Pipelined Adder1/2
  H_p/1 -> Complex to Real-Imag8/1
  H_n/1 -> Complex to Real-Imag1/1
  Constant/1 -> Barrel Shifter/2, Barrel Shifter1/2, Barrel Shifter2/2, Barrel Shifter3/2
  Delay/1 -> Pipelined Adder/1, Barrel Shifter/1
  Delay1/1 -> Pipelined Adder1/1, Barrel Shifter1/1
  Delay2/1 -> Barrel Shifter2/1
  Delay3/1 -> Barrel Shifter3/1
  Pipelined Adder2/1 -> Delay4/1
  Pipelined Adder3/1 -> Delay5/1
  Complex to Real-Imag8/1 -> Delay/1
  Complex to Real-Imag8/2 -> Delay1/1
  Complex to Real-Imag1/1 -> Delay2/1
  Complex to Real-Imag1/2 -> Delay3/1
  Real-Imag to Complex6/1 -> H/1
  Delay4/1 -> Real-Imag to Complex6/1
  Delay5/1 -> Real-Imag to Complex6/2

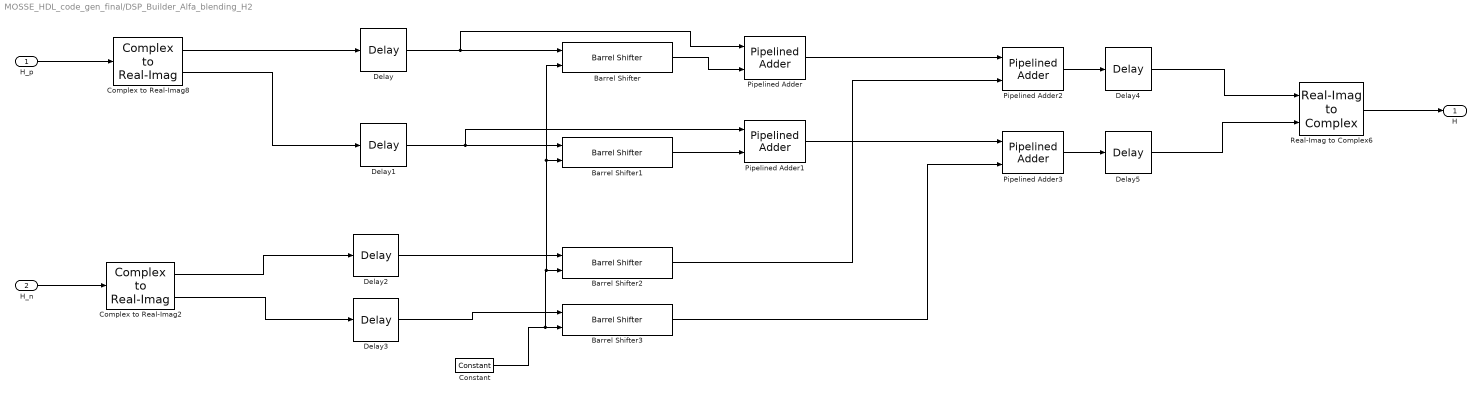
== system MOSSE_HDL_code_gen_final/DSP_Builder_Alfa_blending_H2 ==
  H_p : Inport
  H_n : Inport  Port=2
  Barrel Shifter : allblocks_alteradspbuilder2/Barrel Shifter  BusType=Signed Integer  bwl=32  bwr=8  pipeline=off  infer_distance=off  distance_length=3  ShiftDirection=Shift right  use_ena=off  use_aclr=off  UseDedicatedCircuitry=off  pipeline_display=0  allowFloatingPointOverride=on  logOutputs=off  logFile=E:\Project\AutoTracking\model\MOSSE_work\MOSSE_model\test\tb_MOSSE_HDL_code_gen_final\MOSSE%5FHDL%5Fcode%5Fgen%5Ffinal_DSP%5FBuilder%5FAlfa%5Fblending%5FH2_Barrel+Shifter.fixedpointlog
  Barrel Shifter1 : allblocks_alteradspbuilder2/Barrel Shifter  BusType=Signed Integer  bwl=32  bwr=8  pipeline=off  infer_distance=off  distance_length=3  ShiftDirection=Shift right  use_ena=off  use_aclr=off  UseDedicatedCircuitry=off  pipeline_display=0  allowFloatingPointOverride=on  logOutputs=off  logFile=E:\Project\AutoTracking\model\MOSSE_work\MOSSE_model\test\tb_MOSSE_HDL_code_gen_final\MOSSE%5FHDL%5Fcode%5Fgen%5Ffinal_DSP%5FBuilder%5FAlfa%5Fblending%5FH2_Barrel+Shifter1.fixedpointlog
  Barrel Shifter2 : allblocks_alteradspbuilder2/Barrel Shifter  BusType=Signed Integer  bwl=32  bwr=8  pipeline=off  infer_distance=off  distance_length=3  ShiftDirection=Shift right  use_ena=off  use_aclr=off  UseDedicatedCircuitry=off  pipeline_display=0  allowFloatingPointOverride=on  logOutputs=off  logFile=E:\Project\AutoTracking\model\MOSSE_work\MOSSE_model\test\tb_MOSSE_HDL_code_gen_final\MOSSE%5FHDL%5Fcode%5Fgen%5Ffinal_DSP%5FBuilder%5FAlfa%5Fblending%5FH2_Barrel+Shifter2.fixedpointlog
  Barrel Shifter3 : allblocks_alteradspbuilder2/Barrel Shifter  BusType=Signed Integer  bwl=32  bwr=8  pipeline=off  infer_distance=off  distance_length=3  ShiftDirection=Shift right  use_ena=off  use_aclr=off  UseDedicatedCircuitry=off  pipeline_display=0  allowFloatingPointOverride=on  logOutputs=off  logFile=E:\Project\AutoTracking\model\MOSSE_work\MOSSE_model\test\tb_MOSSE_HDL_code_gen_final\MOSSE%5FHDL%5Fcode%5Fgen%5Ffinal_DSP%5FBuilder%5FAlfa%5Fblending%5FH2_Barrel+Shifter3.fixedpointlog
  Complex to Real-Imag2 : allblocks_alteradspbuilder2/Complex to Real-Imag  BusType=Signed Integer  bwl=32  bwr=0  pipeline_display=0  allowFloatingPointOverride=on  logOutputs=off  logFile=E:\Project\AutoTracking\model\MOSSE_work\MOSSE_model\test\tb_MOSSE_HDL_code_gen_final\MOSSE%5FHDL%5Fcode%5Fgen%5Ffinal_DSP%5FBuilder%5FAlfa%5Fblending%5FH2_Complex+to+Real-Imag2%3A%3Aoutput%5Freal.fixedpointlog,E:\Project\AutoTracking\model\MOSSE_work\MOSSE_model\test\tb_MOSSE_HDL_code_gen_final\MOSSE%5FHDL%5Fcode%5Fgen%5Ffinal_DSP%5FBuilder%5FAlfa%5Fblending%5FH2_Complex+to+Real-Imag2%3A%3Aoutput%5Fimag.fixedpointlog,
  Complex to Real-Imag8 : allblocks_alteradspbuilder2/Complex to Real-Imag  BusType=Signed Integer  bwl=32  bwr=0  pipeline_display=0  allowFloatingPointOverride=on  logOutputs=off  logFile=E:\Project\AutoTracking\model\MOSSE_work\MOSSE_model\test\tb_MOSSE_HDL_code_gen_final\MOSSE%5FHDL%5Fcode%5Fgen%5Ffinal_DSP%5FBuilder%5FAlfa%5Fblending%5FH2_Complex+to+Real-Imag8%3A%3Aoutput%5Freal.fixedpointlog,E:\Project\AutoTracking\model\MOSSE_work\MOSSE_model\test\tb_MOSSE_HDL_code_gen_final\MOSSE%5FHDL%5Fcode%5Fgen%5Ffinal_DSP%5FBuilder%5FAlfa%5Fblending%5FH2_Complex+to+Real-Imag8%3A%3Aoutput%5Fimag.fixedpointlog,
  Constant : allblocks_alteradspbuilder2/Constant  mask_cst=K_shift  BusType=Unsigned Integer  bwl=3  bwr=0  roundMode=Truncate  satMode=Wrap  SpecifyClock=off  allowFloatingPointOverride=on  logOutputs=off  logFile=E:\Project\AutoTracking\model\MOSSE_work\MOSSE_model\test\tb_MOSSE_HDL_code_gen_final\MOSSE%5FHDL%5Fcode%5Fgen%5Ffinal_DSP%5FBuilder%5FAlfa%5Fblending%5FH2_Constant.fixedpointlog
  Delay : allblocks_alteradspbuilder2/Delay  pipeline=1  pipeline_display=1  ClockPhase=1  use_ena=off  use_sclr=off  allowFloatingPointOverride=on  logOutputs=off  logFile=E:\Project\AutoTracking\model\MOSSE_work\MOSSE_model\test\tb_MOSSE_HDL_code_gen_final\MOSSE%5FHDL%5Fcode%5Fgen%5Ffinal_DSP%5FBuilder%5FAlfa%5Fblending%5FH2_Delay.fixedpointlog  use_init=off  reset_value=1
  Delay1 : allblocks_alteradspbuilder2/Delay  pipeline=1  pipeline_display=1  ClockPhase=1  use_ena=off  use_sclr=off  allowFloatingPointOverride=on  logOutputs=off  logFile=E:\Project\AutoTracking\model\MOSSE_work\MOSSE_model\test\tb_MOSSE_HDL_code_gen_final\MOSSE%5FHDL%5Fcode%5Fgen%5Ffinal_DSP%5FBuilder%5FAlfa%5Fblending%5FH2_Delay1.fixedpointlog  use_init=off  reset_value=1
  Delay2 : allblocks_alteradspbuilder2/Delay  pipeline=1  pipeline_display=1  ClockPhase=1  use_ena=off  use_sclr=off  allowFloatingPointOverride=on  logOutputs=off  logFile=E:\Project\AutoTracking\model\MOSSE_work\MOSSE_model\test\tb_MOSSE_HDL_code_gen_final\MOSSE%5FHDL%5Fcode%5Fgen%5Ffinal_DSP%5FBuilder%5FAlfa%5Fblending%5FH2_Delay2.fixedpointlog  use_init=off  reset_value=1
  Delay3 : allblocks_alteradspbuilder2/Delay  pipeline=1  pipeline_display=1  ClockPhase=1  use_ena=off  use_sclr=off  allowFloatingPointOverride=on  logOutputs=off  logFile=E:\Project\AutoTracking\model\MOSSE_work\MOSSE_model\test\tb_MOSSE_HDL_code_gen_final\MOSSE%5FHDL%5Fcode%5Fgen%5Ffinal_DSP%5FBuilder%5FAlfa%5Fblending%5FH2_Delay3.fixedpointlog  use_init=off  reset_value=1
  Delay4 : allblocks_alteradspbuilder2/Delay  pipeline=1  pipeline_display=1  ClockPhase=1  use_ena=off  use_sclr=off  allowFloatingPointOverride=on  logOutputs=off  logFile=E:\Project\AutoTracking\model\MOSSE_work\MOSSE_model\test\tb_MOSSE_HDL_code_gen_final\MOSSE%5FHDL%5Fcode%5Fgen%5Ffinal_DSP%5FBuilder%5FAlfa%5Fblending%5FH2_Delay4.fixedpointlog  use_init=off  reset_value=1
  Delay5 : allblocks_alteradspbuilder2/Delay  pipeline=1  pipeline_display=1  ClockPhase=1  use_ena=off  use_sclr=off  allowFloatingPointOverride=on  logOutputs=off  logFile=E:\Project\AutoTracking\model\MOSSE_work\MOSSE_model\test\tb_MOSSE_HDL_code_gen_final\MOSSE%5FHDL%5Fcode%5Fgen%5Ffinal_DSP%5FBuilder%5FAlfa%5Fblending%5FH2_Delay5.fixedpointlog  use_init=off  reset_value=1
  Pipelined Adder : allblocks_alteradspbuilder2/Pipelined Adder  BusType=Signed Integer  bwl=32  bwr=0  pipeline=0  pipeline_display=0  AddSubDirection=SUB  use_cin=off  use_ovl=off  use_addsub=off  use_ena=off  use_aclr=off  or_aclr_inputs=on
  Pipelined Adder1 : allblocks_alteradspbuilder2/Pipelined Adder  BusType=Signed Integer  bwl=32  bwr=0  pipeline=0  pipeline_display=0  AddSubDirection=SUB  use_cin=off  use_ovl=off  use_addsub=off  use_ena=off  use_aclr=off  or_aclr_inputs=on
  Pipelined Adder2 : allblocks_alteradspbuilder2/Pipelined Adder  BusType=Signed Integer  bwl=32  bwr=0  pipeline=0  pipeline_display=0  AddSubDirection=ADD  use_cin=off  use_ovl=off  use_addsub=off  use_ena=off  use_aclr=off  or_aclr_inputs=on
  Pipelined Adder3 : allblocks_alteradspbuilder2/Pipelined Adder  BusType=Signed Integer  bwl=32  bwr=0  pipeline=0  pipeline_display=0  AddSubDirection=ADD  use_cin=off  use_ovl=off  use_addsub=off  use_ena=off  use_aclr=off  or_aclr_inputs=on
  Real-Imag to Complex6 : allblocks_alteradspbuilder2/Real-Imag to Complex  BusType=Signed Integer  bwl=32  bwr=0  pipeline_display=0  allowFloatingPointOverride=on  logOutputs=off  logFile=E:\Project\AutoTracking\model\MOSSE_work\MOSSE_model\test\tb_MOSSE_HDL_code_gen_final\MOSSE%5FHDL%5Fcode%5Fgen%5Ffinal_DSP%5FBuilder%5FAlfa%5Fblending%5FH2_Real-Imag+to+Complex6.fixedpointlog
  H : Outport
  wires:
  Pipelined Adder/1 -> Pipelined Adder2/1
  Barrel Shifter/1 -> Pipelined Adder/2
  Barrel Shifter2/1 -> Pipelined Adder2/2
  Barrel Shifter3/1 -> Pipelined Adder3/2
  Pipelined Adder1/1 -> Pipelined Adder3/1
  Barrel Shifter1/1 -> Pipelined Adder1/2
  Constant/1 -> Barrel Shifter/2, Barrel Shifter1/2, Barrel Shifter2/2, Barrel Shifter3/2
  Delay/1 -> Pipelined Adder/1, Barrel Shifter/1
  Delay1/1 -> Pipelined Adder1/1, Barrel Shifter1/1
  Delay2/1 -> Barrel Shifter2/1
  Delay3/1 -> Barrel Shifter3/1
  Pipelined Adder2/1 -> Delay4/1
  Pipelined Adder3/1 -> Delay5/1
  H_p/1 -> Complex to Real-Imag8/1
  Complex to Real-Imag8/1 -> Delay/1
  Complex to Real-Imag8/2 -> Delay1/1
  H_n/1 -> Complex to Real-Imag2/1
  Complex to Real-Imag2/1 -> Delay2/1
  Complex to Real-Imag2/2 -> Delay3/1
  Delay4/1 -> Real-Imag to Complex6/1
  Delay5/1 -> Real-Imag to Complex6/2
  Real-Imag to Complex6/1 -> H/1
